simulink model "Vehicle_Model_999_Modular_roll_gradient"  (R2025b)
settings: Solver=ode23tb  StartTime=0.0  StopTime=30  MaxStep=0.001  RelTol=1e-3
values from neighbouring files (symbols this model uses):
  init_r = 0    [Run_this_first.m]
  init_vx = 0    [Run_this_first.m]
  init_vy = 0    [Run_this_first.m]
  Ki_array = zeros(size(Vx_array))    [Torque_vectoring_lookup_table_v3.m]    (also in Torque_vectoring_workspace_lookuptable_v2.m)
  Kp_array = zeros(size(Vx_array))    [Torque_vectoring_workspace_lookuptable_v2.m]
  ku = (lr*m/(cf*(lf+lr))) - (lf*m/(cr*(lf+lr)))    (= -0.000176093739153)    [Torque_vectoring_lookup_table_v3.m]    (also in Torque_vectoring_workspace_lookuptable_v2.m)
  m = Par.m    [LapSim_Endurance_final_ts_v2.m]    (also in Lap_Sim_Final_inverse.m = Par.Mass; Lapsim_Endurance_final_ts.m; New_LapSim_final_ts_v1.m = Par.Mass; Torque_vectoring_lookup_table_v3.m = 270)
  Par = struct()    [Load_vehicle_parameters.m]
  path_Theta = unwrap(atan2(dY, dX))    [New_LapSim_final_ts_v1.m]
  sus_par = struct()    [Load_sus_parameters.m]
  TireData = []    [Lapsim_final_for_app.m]
  V_ref = 45    [Run_this_first.m]
  Vx_array = 1:2:21    [Torque_vectoring_lookup_table_v3.m]    (also in Torque_vectoring_workspace_lookuptable_v2.m = 1:1:21)
undefined symbols (not defined in the file or in its folder): Battery, Brake_Val, ctrl_Brake, ctrl_s, ctrl_Steer, ctrl_Throttle, ctrl_Velocity, HP, Motor, path_X, path_Y, steer_input, Steer_Val, TC_target_slip, Throttle_Val
libraries: simulink x9, autolibshared x3, simulink_extras x2, BatteryEstimators x1
(part 2 of 4)

== system Vehicle_Model_999_Modular_roll_gradient/Vehicle dynamics/Rolling and Drag forces ==
  Aero Drag : MATLAB Function  TreatAsAtomicUnit=on
  Bus Creator : BusCreator  Inputs=3
  Bus Selector : BusSelector  OutputSignals=Fz
  Bus Selector1 : BusSelector  OutputSignals=Steer_FL,Steer_FR
  Bus Selector2 : BusSelector  OutputSignals=Longitudinal_vel,Lateral_vel
  MATLAB Function : MATLAB Function  TreatAsAtomicUnit=on
  Rolling Forces : MATLAB Function  TreatAsAtomicUnit=on
  Terminator : Terminator
  To Workspace : ToWorkspace  Commented=on  VariableName=Dragforce  SaveFormat=Timeseries  SampleTime=-1
  tag scope: Resistive_force_bus=global
  wires:
  Bus Selector1/1 -> Rolling Forces/2(Steer_FL)  "<Steer_FL>"
  Bus Selector2/1 -> Aero Drag/1(vx)  "<Longitudinal_vel>"
  Bus Selector/1 -> Rolling Forces/1(Fz)  "<Fz>"
  Aero Drag/1(B_F_aero) -> MATLAB Function/1(u), Bus Creator/3  "Aero_drag_force"
  Rolling Forces/1(Fx_rr_b) -> Bus Creator/1  "Longitudinal_rolling_resistance"
  Bus Selector1/2 -> Rolling Forces/3(Steer_FR)  "<Steer_FR>"
  Bus Selector2/2 -> Aero Drag/2(vy)  "<Lateral_vel>"
  Rolling Forces/2(Fy_rr_b) -> Bus Creator/2  "Lateral_rolling_resistance"
  Bus Creator/1 -> [Resistive_force_bus]
  MATLAB Function/1(y) -> To Workspace/1, Terminator/1  "Drag_force"
  [Wheel_bus] -> Bus Selector/1
  [Steer_bus] -> Bus Selector1/1
  [chassisbus] -> Bus Selector2/1

== system Vehicle_Model_999_Modular_roll_gradient/Vehicle dynamics/Steering ==
  Bus Selector12 : BusSelector  OutputSignals=Steer_input
  Constant1 : Constant  Value=sus_par.Acc_pct
  Steering Kinematics : Subsystem
  tag scope: Steer_bus=global
  wires:
  Bus Selector12/1 -> Steering Kinematics/1(Steer_Input)  "<Steer_input>"
  Constant1/1 -> Steering Kinematics/2(Ackermann_Pct)
  [Input_bus] -> Bus Selector12/1
  Steering Kinematics/1(Steering Angles) -> [Steer_bus]

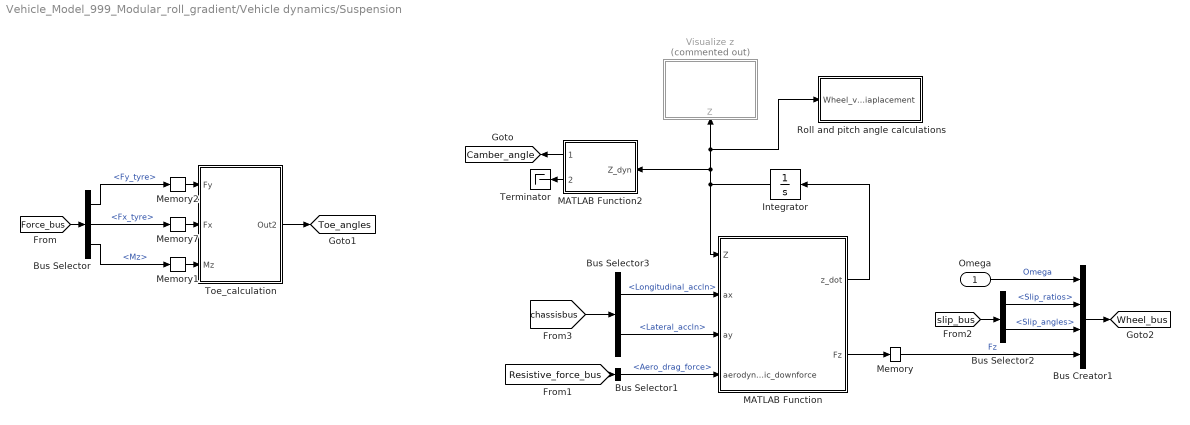
== system Vehicle_Model_999_Modular_roll_gradient/Vehicle dynamics/Suspension ==
  Omega : Inport
  Bus Creator1 : BusCreator  Inputs=4
  Bus Selector : BusSelector  OutputSignals=Fy_tyre,Fx_tyre,Mz
  Bus Selector1 : BusSelector  OutputSignals=Aero_drag_force
  Bus Selector2 : BusSelector  OutputSignals=Slip_ratios,Slip_angles
  Bus Selector3 : BusSelector  OutputSignals=Longitudinal_accln,Lateral_accln
  Integrator : Integrator
  MATLAB Function : MATLAB Function  TreatAsAtomicUnit=on
  MATLAB Function2 : MATLAB Function  TreatAsAtomicUnit=on
  Memory{,1..2,7} (4 alike) : Memory
  Roll and pitch angle calculations : Subsystem
  Terminator : Terminator
  Toe_calculation : Subsystem
  Visualize z : Subsystem  Commented=on
      settings: PortSchema="{\"entries\":[{\"content\":{\"sides\":[{\"content\":{},\"type\":\"ConnectorPlacement.EquallySpacedRectSide\",\"uuid\":\"aa7d9fe9-737c-43ef-afbb-9eca70b49cc7\"},{\"content\":{\"side\":\"RIGHT\"},\"type\":\"ConnectorPlacement.EquallySpacedRectSide\",\"uuid\":\"9d0ef4b4-3bdb-4078-8062-c9c6b9fc0eda\"},{\"content\":{\"side\":\"TOP\"},\"type\":\"ConnectorPlacement.EquallySpacedRectSide\",\"uuid\":\"423cb61c-0fc9-4741-ba0b-eea1eb6461c8\"},{\"content\":{\"connectorIds\":[\"In1\"],\"side\":\"BOTTOM\"},\"type\":\"ConnectorPlacement.EquallySpacedRectSide\",\"uuid\":\"d9a2c6e7-2104-49e5-8c96-ef23060413cc\"}]},\"type\":\"ConnectorPlacement.EquallySpacedConnector\",\"uuid\":\"46e784b7-ddd2-4d2c-b5cf-f45c70590aae\"}],\"packageUris\":[\"http://schema.mathworks.com/mf0/Connector/R2020b\"],\"version\":\"1.0\"}"
  tag scope: Camber_angle=global, Toe_angles=global, Wheel_bus=global
  wires:
  Toe_calculation/1(Out2) -> [Toe_angles]
  Memory7/1 -> Toe_calculation/2(Fx)
  Memory1/1 -> Toe_calculation/3(Mz)
  Memory2/1 -> Toe_calculation/1(Fy)
  Bus Selector/1 -> Memory2/1  "<Fy_tyre>"
  [Force_bus] -> Bus Selector/1
  Bus Selector/2 -> Memory7/1  "<Fx_tyre>"
  Bus Selector/3 -> Memory1/1  "<Mz>"
  Omega/1 -> Bus Creator1/1  "Omega"
  Bus Selector2/2 -> Bus Creator1/3  "<Slip_angles>"
  [chassisbus] -> Bus Selector3/1
  Bus Selector3/1 -> MATLAB Function/2(ax)  "<Longitudinal_accln>"
  Bus Selector2/1 -> Bus Creator1/2  "<Slip_ratios>"
  Bus Selector3/2 -> MATLAB Function/3(ay)  "<Lateral_accln>"
  MATLAB Function/1(z_dot) -> Integrator/1
  Bus Creator1/1 -> [Wheel_bus]
  [slip_bus] -> Bus Selector2/1
  Memory/1 -> Bus Creator1/4  "Fz"
  MATLAB Function/2(Fz) -> Memory/1
  Integrator/1 -> Roll and pitch angle calculations/1(Wheel_vertical_diaplacement), Visualize z/1(Z), MATLAB Function2/1(Z_dyn), MATLAB Function/1(Z)
  MATLAB Function2/1(Camber) -> [Camber_angle]
  MATLAB Function2/2(Camber_gain) -> Terminator/1
  [Resistive_force_bus] -> Bus Selector1/1
  Bus Selector1/1 -> MATLAB Function/4(aerodynamic_downforce)  "<Aero_drag_force>"

== system Vehicle_Model_999_Modular_roll_gradient/Vehicle dynamics/Wheel_dynamics ==
  Bus Selector13 : BusSelector  OutputSignals=Fz
  Bus Selector14 : BusSelector  OutputSignals=Slip_angles
  Bus Selector30 : BusSelector  OutputSignals=Omega
  Rolling Resistance : MATLAB Function  TreatAsAtomicUnit=on
  Wheel Dynamics : Subsystem
  Omega1 : Outport
  wires:
  [Wheel_bus] -> Bus Selector14/1, Bus Selector30/1, Bus Selector13/1
  Bus Selector30/1 -> Rolling Resistance/2(Omega)  "<Omega>"
  Rolling Resistance/1(wFx_rr) -> Wheel Dynamics/1(Fx_rr)
  Bus Selector13/1 -> Rolling Resistance/1(Fz)  "<Fz>"
  Bus Selector14/1 -> Rolling Resistance/3(slip_angles)  "<Slip_angles>"
  Wheel Dynamics/1(Omega) -> Omega1/1

== system Vehicle_Model_999_Modular_roll_gradient/Visualization/Visualize Fx ==
  Fx_tire : Inport
  Demux : Demux
  To Workspace : ToWorkspace  VariableName=Longitudinal_force_fl  SaveFormat=Timeseries  SampleTime=-1
  To Workspace1 : ToWorkspace  VariableName=Longitudinal_force_fr  SaveFormat=Timeseries  SampleTime=-1
  To Workspace2 : ToWorkspace  VariableName=Longitudinal_force_rl  SaveFormat=Timeseries  SampleTime=-1
  To Workspace3 : ToWorkspace  VariableName=Longitudinal_force_rr  SaveFormat=Timeseries  SampleTime=-1
  Visualize_longitudinal_force_tire : Scope  NumInputPorts=4
      settings: ActiveDisplayYMinimum=-1  ActiveDisplayYMaximum=1  DataLoggingVariableName=ScopeData2
  wires:
  Fx_tire/1 -> Demux/1
  Demux/1 -> To Workspace/1, Visualize_longitudinal_force_tire/1  "Longitudinal_force_fl"
  Demux/2 -> To Workspace1/1, Visualize_longitudinal_force_tire/2  "Longitudinal_force_fr"
  Demux/3 -> To Workspace2/1, Visualize_longitudinal_force_tire/3  "Longitudinal_force_rl"
  Demux/4 -> To Workspace3/1, Visualize_longitudinal_force_tire/4  "Longitudinal_force_rr"

== system Vehicle_Model_999_Modular_roll_gradient/Visualization/Visualize Fy ==
  Fy_tire : Inport
  Demux : Demux
  To Workspace1 : ToWorkspace  VariableName=Lateral_force_fl  SaveFormat=Timeseries  SampleTime=-1
  To Workspace2 : ToWorkspace  VariableName=Lateral_force_fr  SaveFormat=Timeseries  SampleTime=-1
  To Workspace3 : ToWorkspace  VariableName=Lateral_force_rl  SaveFormat=Timeseries  SampleTime=-1
  To Workspace4 : ToWorkspace  VariableName=Lateral_force_rr  SaveFormat=Timeseries  SampleTime=-1
  Visualize_lateral_force_tire : Scope  NumInputPorts=4
      settings: ActiveDisplayYMinimum=-1  ActiveDisplayYMaximum=1  DataLoggingVariableName=ScopeData2
  wires:
  Demux/4 -> To Workspace4/1, Visualize_lateral_force_tire/4  "Lateral_force_rr"
  Demux/3 -> To Workspace3/1, Visualize_lateral_force_tire/3  "Lateral_force_rl"
  Demux/2 -> To Workspace2/1, Visualize_lateral_force_tire/2  "Lateral_force_fr"
  Demux/1 -> To Workspace1/1, Visualize_lateral_force_tire/1  "Lateral_force_fl"
  Fy_tire/1 -> Demux/1

== system Vehicle_Model_999_Modular_roll_gradient/Visualization/Visualize Fz ==
  Fz : Inport
  Demux : Demux
  Visualize_Fz : Scope  NumInputPorts=4
      settings: ActiveDisplayYMinimum=-1  ActiveDisplayYMaximum=1  DataLoggingVariableName=ScopeData2
  wires:
  Fz/1 -> Demux/1
  Demux/1 -> Visualize_Fz/1  "Fz_fl"
  Demux/2 -> Visualize_Fz/2  "Fz_fr"
  Demux/3 -> Visualize_Fz/3  "Fz_rl"
  Demux/4 -> Visualize_Fz/4  "Fz_rr"

== system Vehicle_Model_999_Modular_roll_gradient/E-powertrain/Battery Pack/Subsystem ==
  In1 : Inport
  Constant : Constant  Value=0.001
  Switch : Switch  Criteria=u2 > Threshold  SaturateOnIntegerOverflow=off  InputSameDT=off
  Out1 : Outport
  wires:
  In1/1 -> Switch/1, Switch/2
  Constant/1 -> Switch/3
  Switch/1 -> Out1/1

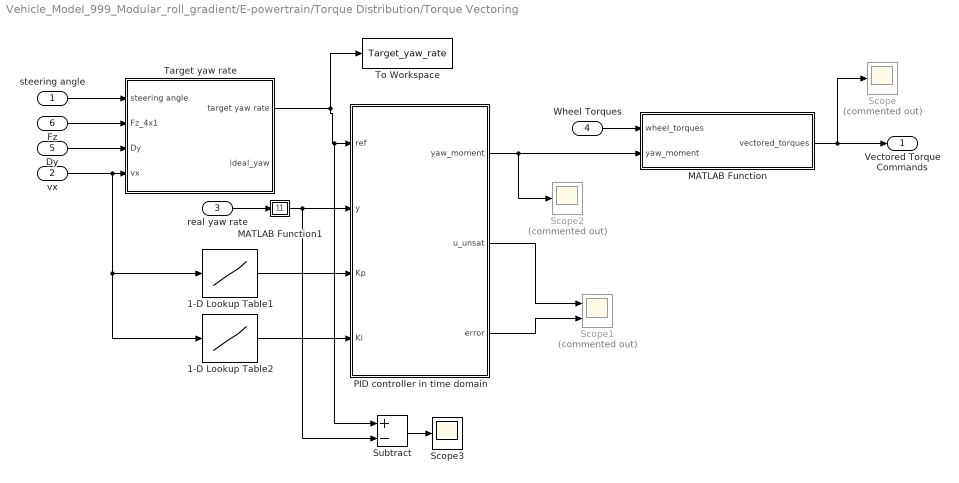
== system Vehicle_Model_999_Modular_roll_gradient/E-powertrain/Torque Distribution/Torque Vectoring ==
  steering angle : Inport
  vx : Inport  Port=2
  real yaw rate : Inport  Port=3
  Wheel Torques : Inport  Port=4
  Dy : Inport  Port=5
  Fz : Inport  Port=6
  1-D Lookup Table1 : Lookup_n-D  NumberOfTableDimensions=1  BreakpointsForDimension1=Vx_array  Table=Kp_array  InternalRulePriority=Speed  RndMeth=Simplest
  1-D Lookup Table2 : Lookup_n-D  NumberOfTableDimensions=1  BreakpointsForDimension1=Vx_array  Table=Ki_array  InternalRulePriority=Speed  RndMeth=Simplest
  MATLAB Function : MATLAB Function  TreatAsAtomicUnit=on
  MATLAB Function1 : MATLAB Function  TreatAsAtomicUnit=on
  PID controller in time domain : MATLAB Function  TreatAsAtomicUnit=on  SystemSampleTime=0.001
  Scope : Scope  Commented=on
      settings: ActiveDisplayYMinimum=-1  ActiveDisplayYMaximum=1  DataLoggingVariableName=ScopeData4
  Scope1 : Scope  Commented=on  NumInputPorts=2
      settings: ActiveDisplayYMinimum=-1  ActiveDisplayYMaximum=1  DataLoggingVariableName=ScopeData15
  Scope2 : Scope  Commented=on
      settings: ActiveDisplayYMinimum=-808.274340814801  ActiveDisplayYMaximum=139.13519650455567  DataLoggingVariableName=ScopeData17
  Scope3 : Scope
      settings: ActiveDisplayYMinimum=-0.85002897198767369  ActiveDisplayYMaximum=1.3983030281875917  DataLoggingVariableName=ScopeData18
  Subtract : Sum  Inputs=+-
  Target yaw rate : Subsystem
  To Workspace : ToWorkspace  VariableName=Target_yaw_rate  SaveFormat=Timeseries  SampleTime=-1
  Vectored Torque Commands : Outport
  wires:
  steering angle/1 -> Target yaw rate/1(steering angle)
  Wheel Torques/1 -> MATLAB Function/1(wheel_torques)
  MATLAB Function/1(vectored_torques) -> Scope/1, Vectored Torque Commands/1
  vx/1 -> 1-D Lookup Table2/1, 1-D Lookup Table1/1, Target yaw rate/4(vx)
  PID controller in time domain/1(yaw_moment) -> Scope2/1, MATLAB Function/2(yaw_moment)
  Fz/1 -> Target yaw rate/2(Fz_4x1)
  Dy/1 -> Target yaw rate/3(Dy)
  real yaw rate/1 -> MATLAB Function1/1(u)
  PID controller in time domain/2(u_unsat) -> Scope1/1
  PID controller in time domain/3(error) -> Scope1/2
  MATLAB Function1/1(y) -> Subtract/2, PID controller in time domain/2(y)
  1-D Lookup Table1/1 -> PID controller in time domain/3(Kp)
  1-D Lookup Table2/1 -> PID controller in time domain/4(Ki)
  Subtract/1 -> Scope3/1
  Target yaw rate/1(target yaw rate) -> Subtract/1, PID controller in time domain/1(ref), To Workspace/1

== system Vehicle_Model_999_Modular_roll_gradient/E-powertrain/Torque Distribution/Traction Control ==
  Wheel Torque : Inport
  Slip Ratios : Inport  Port=2
  vx : Inport  Port=3
  Constant3 : Constant  Value=TC_target_slip
  KD1 : Lookup_n-D  NumberOfTableDimensions=1  BreakpointsForDimension1=[0, 55e-10, 0.0045, 2, 8.5,9]  Table=[0, 0, 0.0014, 0.0109,0,0]  InternalRulePriority=Speed  RndMeth=Simplest
  KI1 : Lookup_n-D  NumberOfTableDimensions=1  BreakpointsForDimension1=[0; 55e-10;0.0045; 2; 8.5]  Table=[0.1; 0.1;700; 500; 450 ]  InternalRulePriority=Speed  RndMeth=Simplest
  KP1 : Lookup_n-D  NumberOfTableDimensions=1  BreakpointsForDimension1=[0; 55e-10; 0.0045; 2; 8.5]  Table=[ 0.5; 0.5; 2.5; 10; 10]  InternalRulePriority=Speed  RndMeth=Simplest
  MATLAB Function1 : MATLAB Function  TreatAsAtomicUnit=on  SystemSampleTime=0.001
  MATLAB Function2 : MATLAB Function  TreatAsAtomicUnit=on
  Traction Controlled Torque : Outport
  wires:
  KD1/1 -> MATLAB Function1/5(Kd)
  KI1/1 -> MATLAB Function1/4(Ki)
  KP1/1 -> MATLAB Function1/3(Kp)
  vx/1 -> KD1/1, KI1/1, KP1/1
  Slip Ratios/1 -> MATLAB Function1/2(lambda_actual)
  Constant3/1 -> MATLAB Function1/1(lambda_ref)
  Wheel Torque/1 -> MATLAB Function2/2(torque_wheel)
  MATLAB Function1/1(throttle_cmd) -> MATLAB Function2/1(torque_pid)
  MATLAB Function2/1(TC_output) -> Traction Controlled Torque/1

== system Vehicle_Model_999_Modular_roll_gradient/E-powertrain/Torque Distribution/is TCS on? ==
  traction_controlled_torque : Inport
  In1 : Inport  Port=2
  TV_T_wheel : Inport  Port=3
  AND : Logic  IconShape=distinctive  AllPortsSameDT=off  OutDataTypeStr=boolean
  NOT : Logic  Operator=NOT  IconShape=distinctive  AllPortsSameDT=off  OutDataTypeStr=boolean
  Switch : Switch  Criteria=u2 > Threshold  SaturateOnIntegerOverflow=off  InputSameDT=off
  torque_output : Outport
  wires:
  Switch/1 -> torque_output/1
  TV_T_wheel/1 -> Switch/3
  traction_controlled_torque/1 -> Switch/1
  In1/1 -> AND/2
  AND/1 -> Switch/2
  [Enable_TV] -> NOT/1
  NOT/1 -> AND/1

== system Vehicle_Model_999_Modular_roll_gradient/E-powertrain/Torque Distribution/is TV on? ==
  vectored_torque : Inport
  In1 : Inport  Port=2
  wheel_torque : Inport  Port=3
  AND : Logic  IconShape=distinctive  AllPortsSameDT=off  OutDataTypeStr=boolean
  Switch : Switch  Criteria=u2 > Threshold  SaturateOnIntegerOverflow=off  InputSameDT=off
  torque_output : Outport
  wires:
  wheel_torque/1 -> Switch/3
  vectored_torque/1 -> Switch/1
  Switch/1 -> torque_output/1
  AND/1 -> Switch/2
  In1/1 -> AND/2
  [Enable_TV] -> AND/1

== system Vehicle_Model_999_Modular_roll_gradient/Inputs/Brake_input_selector/Brake Variant Subsystem ==
  brake_sim : Inport
  vel : Inport  Port=2
  GGV : Subsystem  VariantControl=Mode_ggv
  Sideslip_vs_curvature_cst_accln : Subsystem  VariantControl=Mode_sideslip_vs_curvature_cst_accln
  Simulink : Subsystem  VariantControl=Mode_simulink
  curvature vs steer_angle : Subsystem  VariantControl=Mode_curvature_vs_steer
  sideslip_vs_curvature : Subsystem  VariantControl=Mode_sideslip_vs_curvature
  steerdiff_vs_ay : Subsystem  VariantControl=Mode_steerdiff_vs_ay
  timeseries : Subsystem  VariantControl=Mode_timeseries
  brake_input : Outport
  accln : Outport  Port=2

== system Vehicle_Model_999_Modular_roll_gradient/Inputs/Subsystem/Triggered Subsystem ==
  In1 : Inport
  Trigger : TriggerPort  VariantControl=(inherit)
  Out1 : Outport
  wires:
  In1/1 -> Out1/1

== system Vehicle_Model_999_Modular_roll_gradient/Inputs/Subsystem/Triggered Subsystem1 ==
  In1 : Inport
  Trigger : TriggerPort  VariantControl=(inherit)
  Out1 : Outport
  wires:
  In1/1 -> Out1/1

== system Vehicle_Model_999_Modular_roll_gradient/Inputs/Subsystem/Triggered Subsystem2 ==
  In1 : Inport
  Trigger : TriggerPort  VariantControl=(inherit)
  Out1 : Outport
  wires:
  In1/1 -> Out1/1

== system Vehicle_Model_999_Modular_roll_gradient/Inputs/Throttle_input_selector/Throttle Variant Subsystem ==
  accln : Inport
  accln_input_for_map1 : Inport  Port=2
  GGV : Subsystem  VariantControl=Mode_ggv
  Simulink : Subsystem  VariantControl=Mode_simulink
  Timeseries : Subsystem  VariantControl=Mode_timeseries
  curvature vs steer : Subsystem  VariantControl=Mode_curvature_vs_steer
  sideslip_vs_curvature : Subsystem  VariantControl=Mode_sideslip_vs_curvature
  sideslip_vs_curvature_cst_accln : Subsystem  VariantControl=Mode_sideslip_vs_curvature_cst_accln
  steerdiff_vs_ay : Subsystem  VariantControl=Mode_steerdiff_vs_ay
  throttle : Outport

== system Vehicle_Model_999_Modular_roll_gradient/Inputs/steer_input_selector/Steering Variant Subsystem ==
  In1 : Inport
  GGV : Subsystem  VariantControl=Mode_ggv
  Simulink : Subsystem  VariantControl=Mode_simulink
  Timeseries : Subsystem  VariantControl=Mode_timeseries
  curvature_vs_steering_angle : Subsystem  VariantControl=Mode_curvature_vs_steer
  sideslip_vs_curvature_1 : Subsystem  VariantControl=Mode_sideslip_vs_curvature
  sideslip_vs_curvature_constant_lat_accln : Subsystem  VariantControl=Mode_sideslip_vs_curvature_cst_accln
  steerdiff_vs_ay : Subsystem  VariantControl=Mode_steerdiff_vs_ay
  Steer Input : Outport

== system Vehicle_Model_999_Modular_roll_gradient/Vehicle dynamics/Force and Torque Equilibrium/Subsystem ==
  In1 : Inport
  Clock : Clock
  Compare To Constant : simulink/Logic and Bit Operations/Compare To Constant  relop=>=  const=75  OutDataTypeStr=boolean
  Detect Rise Positive : simulink/Logic and Bit Operations/Detect Rise Positive  vinit=0  OutDataTypeStr=boolean
  Triggered Subsystem : Subsystem  TreatAsAtomicUnit=on
  Out1 : Outport
  wires:
  In1/1 -> Compare To Constant/1
  Detect Rise Positive/1 -> Triggered Subsystem/Trigger
  Clock/1 -> Triggered Subsystem/1(In1)
  Triggered Subsystem/1(Out1) -> Out1/1
  Compare To Constant/1 -> Detect Rise Positive/1

== system Vehicle_Model_999_Modular_roll_gradient/Vehicle dynamics/Force and Torque Equilibrium/Subsystem1 ==
  In1 : Inport
  Constant : Constant  Value=0.001
  Switch : Switch  Criteria=u2 > Threshold  SaturateOnIntegerOverflow=off  InputSameDT=off
  Out1 : Outport
  wires:
  In1/1 -> Switch/1, Switch/2
  Constant/1 -> Switch/3
  Switch/1 -> Out1/1

== system Vehicle_Model_999_Modular_roll_gradient/Vehicle dynamics/Force and Torque Equilibrium/Visualize Fx ==
  Fx_body : Inport
  Demux : Demux
  To Workspace : ToWorkspace  VariableName=Longitudinal_force_body_fl  SaveFormat=Timeseries  SampleTime=-1
  To Workspace1 : ToWorkspace  VariableName=Longitudinal_force_body_fr  SaveFormat=Timeseries  SampleTime=-1
  To Workspace2 : ToWorkspace  VariableName=Longitudinal_force_body_rl  SaveFormat=Timeseries  SampleTime=-1
  To Workspace3 : ToWorkspace  VariableName=Longitudinal_force_body_rr  SaveFormat=Timeseries  SampleTime=-1
  Visualize_longitudinal_force_body : Scope  NumInputPorts=4
      settings: ActiveDisplayYMinimum=-1  ActiveDisplayYMaximum=1  DataLoggingVariableName=ScopeData2
  wires:
  Fx_body/1 -> Demux/1
  Demux/1 -> To Workspace/1, Visualize_longitudinal_force_body/1  "Longitudinal_force_fl"
  Demux/2 -> To Workspace1/1, Visualize_longitudinal_force_body/2  "Longitudinal_force_fr"
  Demux/3 -> To Workspace2/1, Visualize_longitudinal_force_body/3  "Longitudinal_force_rl"
  Demux/4 -> To Workspace3/1, Visualize_longitudinal_force_body/4  "Longitudinal_force_rr"

== system Vehicle_Model_999_Modular_roll_gradient/Vehicle dynamics/Force and Torque Equilibrium/Visualize Fy ==
  Fy_tire : Inport
  Demux : Demux
  To Workspace1 : ToWorkspace  VariableName=Lateral_force_body_fl  SaveFormat=Timeseries  SampleTime=-1
  To Workspace2 : ToWorkspace  VariableName=Lateral_force_body_fr  SaveFormat=Timeseries  SampleTime=-1
  To Workspace3 : ToWorkspace  VariableName=Lateral_force_body_rl  SaveFormat=Timeseries  SampleTime=-1
  To Workspace4 : ToWorkspace  VariableName=Lateral_force_body_rr  SaveFormat=Timeseries  SampleTime=-1
  Visualize_lateral_force_body : Scope  NumInputPorts=4
      settings: ActiveDisplayYMinimum=-1  ActiveDisplayYMaximum=1  DataLoggingVariableName=ScopeData2
  wires:
  Demux/4 -> To Workspace4/1, Visualize_lateral_force_body/4  "Lateral_force_rr"
  Demux/3 -> To Workspace3/1, Visualize_lateral_force_body/3  "Lateral_force_rl"
  Demux/2 -> To Workspace2/1, Visualize_lateral_force_body/2  "Lateral_force_fr"
  Demux/1 -> To Workspace1/1, Visualize_lateral_force_body/1  "Lateral_force_fl"
  Fy_tire/1 -> Demux/1

== system Vehicle_Model_999_Modular_roll_gradient/Vehicle dynamics/Fx, Fy calculations/Slip_angle_calculation ==
  Bus Selector25 : BusSelector  OutputSignals=Longitudinal_vel
  Bus Selector26 : BusSelector  OutputSignals=Lateral_vel
  Bus Selector27 : BusSelector  OutputSignals=Yaw_rate
  Bus Selector28 : BusSelector  OutputSignals=Steer_FL
  Bus Selector29 : BusSelector  OutputSignals=Steer_FR
  Slip Angles : MATLAB Function  TreatAsAtomicUnit=on
  Subsystem : Subsystem
  Visualize Slip_angle : Subsystem  Commented=on
  effective_slip_angle : Outport
  wires:
  Bus Selector26/1 -> Slip Angles/2(Lateral_vel)  "<Lateral_vel>"
  Bus Selector27/1 -> Slip Angles/3(yawrate)  "<Yaw_rate>"
  [Steer_bus] -> Bus Selector29/1, Bus Selector28/1
  [chassisbus] -> Bus Selector27/1, Bus Selector26/1, Bus Selector25/1
  Bus Selector25/1 -> Slip Angles/1(Longitudinal_vel)  "<Longitudinal_vel>"
  Slip Angles/1(slip_angles) -> Subsystem/2(slip_angles)
  Bus Selector28/1 -> Slip Angles/4(Steer_FL)  "<Steer_FL>"
  Bus Selector29/1 -> Slip Angles/5(Steer_FR)  "<Steer_FR>"
  Subsystem/1(slip_ratio) -> Visualize Slip_angle/1(slip_angle), effective_slip_angle/1  "effective_slip_angle"
  [Toe_angles] -> Subsystem/1(toe)

== system Vehicle_Model_999_Modular_roll_gradient/Vehicle dynamics/Fx, Fy calculations/Slip_ratio_calculation ==
  Bus Selector21 : BusSelector  OutputSignals=Longitudinal_vel
  Bus Selector22 : BusSelector  OutputSignals=Yaw_rate
  Bus Selector23 : BusSelector  OutputSignals=Omega
  Bus Selector24 : BusSelector  OutputSignals=Lateral_vel
  Bus Selector32 : BusSelector  OutputSignals=Steer_FL
  Bus Selector33 : BusSelector  OutputSignals=Steer_FR
  Visualize Slip_ratios : Subsystem  Commented=on
  slip ratios : MATLAB Function  TreatAsAtomicUnit=on
  slip_ratios : Outport
  wires:
  [Steer_bus] -> Bus Selector32/1, Bus Selector33/1
  Bus Selector21/1 -> slip ratios/1(Vx)  "<Longitudinal_vel>"
  Bus Selector23/1 -> slip ratios/4(Omega)  "<Omega>"
  Bus Selector32/1 -> slip ratios/5(Steer_FL)  "<Steer_FL>"
  [chassisbus] -> Bus Selector22/1, Bus Selector24/1, Bus Selector21/1
  Bus Selector22/1 -> slip ratios/3(yawrate)  "<Yaw_rate>"
  Bus Selector33/1 -> slip ratios/6(Steer_FR)  "<Steer_FR>"
  Bus Selector24/1 -> slip ratios/2(Vy)  "<Lateral_vel>"
  [Wheel_bus] -> Bus Selector23/1
  slip ratios/1(slip_ratios) -> Visualize Slip_ratios/1(slip_ratio), slip_ratios/1  "slip_ratios"

== system Vehicle_Model_999_Modular_roll_gradient/Vehicle dynamics/Fx, Fy calculations/Tyre_relaxation ==
  Fx_ss : Inport
  Bus Selector : BusSelector  OutputSignals=Longitudinal_vel
  Integrator : Integrator
  MATLAB Function : MATLAB Function  TreatAsAtomicUnit=on
  Fx_w : Outport
  wires:
  Fx_ss/1 -> MATLAB Function/1(Fx_ss)
  MATLAB Function/1(Fx_dot) -> Integrator/1
  Integrator/1 -> Fx_w/1, MATLAB Function/2(Fx_act)
  Bus Selector/1 -> MATLAB Function/3(Vx)  "<Longitudinal_vel>"
  [chassisbus] -> Bus Selector/1

== system Vehicle_Model_999_Modular_roll_gradient/Vehicle dynamics/Fx, Fy calculations/Visualise_Fy_B ==
  Fy_B : Inport
  MATLAB Function : MATLAB Function  TreatAsAtomicUnit=on
  Visualise Fy_B : Scope  Commented=on  NumInputPorts=4
  wires:
  Fy_B/1 -> MATLAB Function/1(Fy_tire)
  MATLAB Function/2(Fy_B_fr) -> Visualise Fy_B/2  "Fy_B_fr"
  MATLAB Function/4(Fy_B_rr) -> Visualise Fy_B/4  "Fy_B_rr"
  MATLAB Function/1(Fy_B_fl) -> Visualise Fy_B/1  "Fy_B_fl"
  MATLAB Function/3(Fy_B_rl) -> Visualise Fy_B/3  "Fy_B_rl"

== system Vehicle_Model_999_Modular_roll_gradient/Vehicle dynamics/Fx, Fy calculations/Visualiser ==
  mz : Inport
  mu_x : Inport  Port=2
  mu_y : Inport  Port=3
  Demux : Demux
  Demux1 : Demux
  Demux2 : Demux
  Scope : Scope  NumInputPorts=4
  Scope1 : Scope  NumInputPorts=4
  Scope2 : Scope  NumInputPorts=4
  wires:
  mz/1 -> Demux/1
  Demux/1 -> Scope/1
  Demux/2 -> Scope/2
  Demux/3 -> Scope/3
  Demux/4 -> Scope/4
  Demux1/3 -> Scope1/3
  Demux1/2 -> Scope1/2
  mu_x/1 -> Demux1/1
  Demux1/1 -> Scope1/1
  Demux1/4 -> Scope1/4
  Demux2/3 -> Scope2/3
  Demux2/2 -> Scope2/2
  mu_y/1 -> Demux2/1
  Demux2/1 -> Scope2/1
  Demux2/4 -> Scope2/4

== system Vehicle_Model_999_Modular_roll_gradient/Vehicle dynamics/Fx, Fy calculations with grip limit/Grip_limit ==
  Fx : Inport
  Fy_tyre : Inport  Port=2
  Bus Selector2 : BusSelector  OutputSignals=Dx,Dy
  Bus Selector3 : BusSelector  OutputSignals=Longitudinal_disp
  MATLAB Function1 : MATLAB Function  TreatAsAtomicUnit=on
  Fx_new : Outport
  Fy_new : Outport  Port=2
  wires:
  Bus Selector2/2 -> MATLAB Function1/4(Dy)  "<Dy>"
  Bus Selector3/1 -> MATLAB Function1/5(s)  "<Longitudinal_disp>"
  Bus Selector2/1 -> MATLAB Function1/3(Dx)  "<Dx>"
  [chassisbus] -> Bus Selector3/1
  [Force_bus] -> Bus Selector2/1
  MATLAB Function1/1(Fx_new) -> Fx_new/1
  Fy_tyre/1 -> MATLAB Function1/2(Fy)
  Fx/1 -> MATLAB Function1/1(Fx)
  MATLAB Function1/2(Fy_new) -> Fy_new/1

== system Vehicle_Model_999_Modular_roll_gradient/Vehicle dynamics/Fx, Fy calculations with grip limit/Slip_angle_calculation ==
  Bus Selector25 : BusSelector  OutputSignals=Longitudinal_vel
  Bus Selector26 : BusSelector  OutputSignals=Lateral_vel
  Bus Selector27 : BusSelector  OutputSignals=Yaw_rate
  Bus Selector28 : BusSelector  OutputSignals=Steer_FL
  Bus Selector29 : BusSelector  OutputSignals=Steer_FR
  Slip Angles : MATLAB Function  TreatAsAtomicUnit=on
  Subsystem : Subsystem
  Visualize Slip_angle : Subsystem  Commented=on
  effective_slip_angle : Outport
  wires:
  [Toe_angles] -> Subsystem/1(toe)
  Subsystem/1(slip_ratio) -> effective_slip_angle/1, Visualize Slip_angle/1(slip_angle)  "effective_slip_angle"
  Bus Selector29/1 -> Slip Angles/5(Steer_FR)  "<Steer_FR>"
  Bus Selector28/1 -> Slip Angles/4(Steer_FL)  "<Steer_FL>"
  Slip Angles/1(slip_angles) -> Subsystem/2(slip_angles)
  Bus Selector25/1 -> Slip Angles/1(Longitudinal_vel)  "<Longitudinal_vel>"
  [chassisbus] -> Bus Selector25/1, Bus Selector26/1, Bus Selector27/1
  [Steer_bus] -> Bus Selector28/1, Bus Selector29/1
  Bus Selector27/1 -> Slip Angles/3(yawrate)  "<Yaw_rate>"
  Bus Selector26/1 -> Slip Angles/2(Lateral_vel)  "<Lateral_vel>"

== system Vehicle_Model_999_Modular_roll_gradient/Vehicle dynamics/Fx, Fy calculations with grip limit/Slip_ratio_calculation ==
  Bus Selector21 : BusSelector  OutputSignals=Longitudinal_vel
  Bus Selector22 : BusSelector  OutputSignals=Yaw_rate
  Bus Selector23 : BusSelector  OutputSignals=Omega
  Bus Selector24 : BusSelector  OutputSignals=Lateral_vel
  Bus Selector32 : BusSelector  OutputSignals=Steer_FL
  Bus Selector33 : BusSelector  OutputSignals=Steer_FR
  Visualize Slip_ratios : Subsystem  Commented=on
  slip ratios : MATLAB Function  TreatAsAtomicUnit=on
  slip_ratios : Outport
  wires:
  slip ratios/1(slip_ratios) -> slip_ratios/1, Visualize Slip_ratios/1(slip_ratio)  "slip_ratios"
  [Wheel_bus] -> Bus Selector23/1
  Bus Selector24/1 -> slip ratios/2(Vy)  "<Lateral_vel>"
  Bus Selector33/1 -> slip ratios/6(Steer_FR)  "<Steer_FR>"
  Bus Selector22/1 -> slip ratios/3(yawrate)  "<Yaw_rate>"
  [chassisbus] -> Bus Selector21/1, Bus Selector24/1, Bus Selector22/1
  Bus Selector32/1 -> slip ratios/5(Steer_FL)  "<Steer_FL>"
  Bus Selector23/1 -> slip ratios/4(Omega)  "<Omega>"
  Bus Selector21/1 -> slip ratios/1(Vx)  "<Longitudinal_vel>"
  [Steer_bus] -> Bus Selector33/1, Bus Selector32/1

== system Vehicle_Model_999_Modular_roll_gradient/Vehicle dynamics/Fx, Fy calculations with grip limit/Tyre_relaxation ==
  Fx_ss : Inport
  Bus Selector : BusSelector  OutputSignals=Longitudinal_vel
  Integrator : Integrator
  MATLAB Function : MATLAB Function  TreatAsAtomicUnit=on
  Fx_w : Outport
  wires:
  [chassisbus] -> Bus Selector/1
  Bus Selector/1 -> MATLAB Function/3(Vx)  "<Longitudinal_vel>"
  Integrator/1 -> MATLAB Function/2(Fx_act), Fx_w/1
  MATLAB Function/1(Fx_dot) -> Integrator/1
  Fx_ss/1 -> MATLAB Function/1(Fx_ss)

== system Vehicle_Model_999_Modular_roll_gradient/Vehicle dynamics/Fx, Fy calculations with grip limit/Visualise_Fy_B ==
  Fy_B : Inport
  MATLAB Function : MATLAB Function  TreatAsAtomicUnit=on
  Visualise Fy_B : Scope  Commented=on  NumInputPorts=4
  wires:
  MATLAB Function/3(Fy_B_rl) -> Visualise Fy_B/3  "Fy_B_rl"
  MATLAB Function/1(Fy_B_fl) -> Visualise Fy_B/1  "Fy_B_fl"
  MATLAB Function/4(Fy_B_rr) -> Visualise Fy_B/4  "Fy_B_rr"
  MATLAB Function/2(Fy_B_fr) -> Visualise Fy_B/2  "Fy_B_fr"
  Fy_B/1 -> MATLAB Function/1(Fy_tire)

== system Vehicle_Model_999_Modular_roll_gradient/Vehicle dynamics/Fx, Fy calculations with grip limit/Visualiser ==
  mz : Inport
  mu_x : Inport  Port=2
  mu_y : Inport  Port=3
  Demux : Demux
  Demux1 : Demux
  Demux2 : Demux
  Scope : Scope  NumInputPorts=4
  Scope1 : Scope  NumInputPorts=4
  Scope2 : Scope  NumInputPorts=4
  wires:
  Demux2/4 -> Scope2/4
  Demux2/1 -> Scope2/1
  mu_y/1 -> Demux2/1
  Demux2/2 -> Scope2/2
  Demux2/3 -> Scope2/3
  Demux1/4 -> Scope1/4
  Demux1/1 -> Scope1/1
  mu_x/1 -> Demux1/1
  Demux1/2 -> Scope1/2
  Demux1/3 -> Scope1/3
  Demux/4 -> Scope/4
  Demux/3 -> Scope/3
  Demux/2 -> Scope/2
  Demux/1 -> Scope/1
  mz/1 -> Demux/1

== system Vehicle_Model_999_Modular_roll_gradient/Vehicle dynamics/Steering/Steering Kinematics ==
  Steer_Input : Inport
  Ackermann_Pct : Inport  Port=2
  Bus Creator1 : BusCreator  Inputs=2
  Steering Kinematics : MATLAB Function  TreatAsAtomicUnit=on
  To Workspace : ToWorkspace  VariableName=steer_L  SaveFormat=Timeseries  SampleTime=-1
  To Workspace1 : ToWorkspace  VariableName=steer_R  SaveFormat=Timeseries  SampleTime=-1
  Steering Angles : Outport
  wires:
  Steering Kinematics/1(Steer_FL) -> To Workspace/1, Bus Creator1/1  "Steer_FL"
  Steer_Input/1 -> Steering Kinematics/1(Steer_Input)
  Steering Kinematics/2(Steer_FR) -> To Workspace1/1, Bus Creator1/2  "Steer_FR"
  Ackermann_Pct/1 -> Steering Kinematics/2(Ackermann_Pct)
  Bus Creator1/1 -> Steering Angles/1

== system Vehicle_Model_999_Modular_roll_gradient/Vehicle dynamics/Suspension/Roll and pitch angle calculations ==
  Wheel_vertical_diaplacement : Inport
  Gain : Gain  Gain=180/pi
  Gain1 : Gain  Gain=180/pi
  Pitch_angle_calcualtions : MATLAB Function  TreatAsAtomicUnit=on
  Roll_angle_calulations : MATLAB Function  TreatAsAtomicUnit=on
  To Workspace : ToWorkspace  VariableName=roll_angle  SaveFormat=Timeseries  SampleTime=-1
  Visualize pitch angle : Scope
      settings: ActiveDisplayYMinimum=-0.081148408984306142  ActiveDisplayYMaximum=0.65312774588570066  DataLoggingVariableName=ScopeData5
  Visualize roll angle : Scope
      settings: ActiveDisplayYMinimum=-1  ActiveDisplayYMaximum=1  DataLoggingVariableName=ScopeData6
  wires:
  Wheel_vertical_diaplacement/1 -> Pitch_angle_calcualtions/1(z_wheel), Roll_angle_calulations/1(z_wheel)
  Pitch_angle_calcualtions/1(Pitch_angle) -> Gain/1
  Roll_angle_calulations/1(Roll_angle) -> Gain1/1
  Gain/1 -> Visualize pitch angle/1
  Gain1/1 -> To Workspace/1, Visualize roll angle/1

== system Vehicle_Model_999_Modular_roll_gradient/Vehicle dynamics/Suspension/Toe_calculation ==
  Fy : Inport
  Fx : Inport  Port=2
  Mz : Inport  Port=3
  Mux1 : Mux
  toe_fl1 : MATLAB Function  TreatAsAtomicUnit=on
  Out2 : Outport
  wires:
  Mux1/1 -> Out2/1
  Mz/1 -> toe_fl1/3(Mz)
  Fx/1 -> toe_fl1/2(Fx_tire)
  Fy/1 -> toe_fl1/1(Fy_tire)
  toe_fl1/1(Toe_fl) -> Mux1/1
  toe_fl1/2(Toe_fr) -> Mux1/2
  toe_fl1/3(Toe_rl) -> Mux1/3
  toe_fl1/4(Toe_rr) -> Mux1/4

== system Vehicle_Model_999_Modular_roll_gradient/Vehicle dynamics/Suspension/Visualize z ==
  Z : Inport
  Demux : Demux
  Visualize_wheel_vertical_displacement : Scope  NumInputPorts=4
      settings: ActiveDisplayYMinimum=-0.0083526738061748679  ActiveDisplayYMaximum=0.0034975178963681597  DataLoggingVariableName=ScopeData2
  wires:
  Z/1 -> Demux/1
  Demux/1 -> Visualize_wheel_vertical_displacement/1  "z_fl"
  Demux/2 -> Visualize_wheel_vertical_displacement/2  "z_fr"
  Demux/3 -> Visualize_wheel_vertical_displacement/3  "z_rl"
  Demux/4 -> Visualize_wheel_vertical_displacement/4  "z_rr"

== system Vehicle_Model_999_Modular_roll_gradient/Vehicle dynamics/Wheel_dynamics/Wheel Dynamics ==
  Fx_rr : Inport
  Bus Selector8 : BusSelector  OutputSignals=Fx_tyre
  Integrator : Integrator  InitialCondition=init_vx/Par.R0  LimitOutput=on  UpperSaturationLimit=1e6
  MATLAB Function : MATLAB Function  TreatAsAtomicUnit=on
  Saturation : Saturate  UpperLimit=Motor.n_max*2*pi/(60*10.05)  LowerLimit=0
  Omega : Outport
  wires:
  [Torque_inputs] -> MATLAB Function/1(T_in)
  Fx_rr/1 -> MATLAB Function/2(Fx_rr)
  Integrator/1 -> Saturation/1
  MATLAB Function/1(Omega_dot) -> Integrator/1
  [Force_bus] -> Bus Selector8/1
  Bus Selector8/1 -> MATLAB Function/3(Fx_tire)  "<Fx_tyre>"
  Saturation/1 -> Omega/1, MATLAB Function/4(Omega)

== system Vehicle_Model_999_Modular_roll_gradient/E-powertrain/Torque Distribution/Torque Vectoring/Target yaw rate ==
  steering angle : Inport
  Fz_4x1 : Inport  Port=2
  Dy : Inport  Port=3
  vx : Inport  Port=4
  MATLAB Function : MATLAB Function  TreatAsAtomicUnit=on
  target yaw rate : Outport
  ideal_yaw : Outport  Port=2
  tag scope: Enable_TV=global
  wires:
  vx/1 -> MATLAB Function/1(vx)
  Fz_4x1/1 -> MATLAB Function/4(Fz)
  Dy/1 -> MATLAB Function/3(Dy)
  steering angle/1 -> MATLAB Function/2(delta)
  MATLAB Function/1(target_yaw) -> target yaw rate/1
  MATLAB Function/2(ideal_yaw) -> ideal_yaw/1
  MATLAB Function/3(tv_enable) -> [Enable_TV]

== system Vehicle_Model_999_Modular_roll_gradient/Inputs/Brake_input_selector/Brake Variant Subsystem/GGV ==
  Constant : Constant  Value=Brake_Val
  brake_input : Outport
  wires:
  Constant/1 -> brake_input/1

== system Vehicle_Model_999_Modular_roll_gradient/Inputs/Brake_input_selector/Brake Variant Subsystem/Sideslip_vs_curvature_cst_accln ==
  vel : Inport
  Constant : Constant  Value=10
  Constant3 : Constant  Value=0
  Longitudinal Driver : autolibshared/Longitudinal Driver  extAccelOvr=off  extDecelOvr=off  extAccelHld=off  extDecelHld=off  extAccelZero=off  extDecelZero=off  cntrlType=PI  shftType=None  velUnits=m/s  gearOut=off  Kp=10  Ki=5  Kff=.1  Kg=0  VehVelVec=[0 100]  KffVec=[.1 .1]  KpVec=[10 10]  KiVec=[5 5]  KgVec=[0 0]  m=1500  Kpt=3000  tau=.1  L=2  aR=200  bR=2.5  cR=.5  g=9.81  vnom=5  Kaw=1  tauerr=.01  tauPt=2  GearInit=0  tShift=.1  pdlVec=[0.1 0.4 0.5 0.9]  upShftTbl=[-1 12.9375 26.4375 39.9375 51.18749999999999 62.4375 72.84375 83.25;-1 16.3125 29.8125 43.3125 54.5624 65.8125 76.78125 87.75;-1 19.6875 33.1875 46.68749999999999 57.9375 69.1875 80.71875 92.25;-1 33 52.5 77.25 100.5 138.75 161.875 185]  dwnShftTbl=[1 9.5625 23.0625 36.5625 47.8125 59.0625 68.90625 78.75;1 12.9375 26.4375 39.9375 51.18749999999999 62.4375 72.84375 83.25;1 16.3125 29.8125 43.3125 54.562499 65.8125 76.78125 87.75;1 19.6875 33.1875 46.68749999999999 57.9375 69.1875 80.71875 92.25]  tClutch=.5  tRev=.5  tPark=120  aMode=2  UpGearVec="[0  1  2  3  4  5  6  7]"  DownGearVec="[1  2  3  4  5  6  7  8]"
      settings: LibrarySourceBlock=vehdynlibdriver/Longitudinal Driver
  Terminator1 : Terminator
  brake_input : Outport
  accln : Outport  Port=2
  wires:
  Constant3/1 -> Longitudinal Driver/3
  Constant/1 -> Longitudinal Driver/1
  Longitudinal Driver/1 -> Terminator1/1
  Longitudinal Driver/2 -> accln/1
  Longitudinal Driver/3 -> brake_input/1
  vel/1 -> Longitudinal Driver/2

== system Vehicle_Model_999_Modular_roll_gradient/Inputs/Brake_input_selector/Brake Variant Subsystem/Simulink ==
  brake_sim : Inport
  brake_input : Outport
  wires:
  brake_sim/1 -> brake_input/1

== system Vehicle_Model_999_Modular_roll_gradient/Inputs/Brake_input_selector/Brake Variant Subsystem/curvature vs steer_angle ==
  vel : Inport
  Constant : Constant  Value=V_ref
  Constant3 : Constant  Value=0
  Longitudinal Driver : autolibshared/Longitudinal Driver  extAccelOvr=off  extDecelOvr=off  extAccelHld=off  extDecelHld=off  extAccelZero=off  extDecelZero=off  cntrlType=PI  shftType=None  velUnits=m/s  gearOut=off  Kp=10  Ki=5  Kff=.1  Kg=0  VehVelVec=[0 100]  KffVec=[.1 .1]  KpVec=[10 10]  KiVec=[5 5]  KgVec=[0 0]  m=1500  Kpt=3000  tau=.1  L=2  aR=200  bR=2.5  cR=.5  g=9.81  vnom=5  Kaw=1  tauerr=.01  tauPt=2  GearInit=0  tShift=.1  pdlVec=[0.1 0.4 0.5 0.9]  upShftTbl=[-1 12.9375 26.4375 39.9375 51.18749999999999 62.4375 72.84375 83.25;-1 16.3125 29.8125 43.3125 54.5624 65.8125 76.78125 87.75;-1 19.6875 33.1875 46.68749999999999 57.9375 69.1875 80.71875 92.25;-1 33 52.5 77.25 100.5 138.75 161.875 185]  dwnShftTbl=[1 9.5625 23.0625 36.5625 47.8125 59.0625 68.90625 78.75;1 12.9375 26.4375 39.9375 51.18749999999999 62.4375 72.84375 83.25;1 16.3125 29.8125 43.3125 54.562499 65.8125 76.78125 87.75;1 19.6875 33.1875 46.68749999999999 57.9375 69.1875 80.71875 92.25]  tClutch=.5  tRev=.5  tPark=120  aMode=2  UpGearVec="[0  1  2  3  4  5  6  7]"  DownGearVec="[1  2  3  4  5  6  7  8]"
      settings: LibrarySourceBlock=vehdynlibdriver/Longitudinal Driver
  Terminator : Terminator
  brake_input : Outport
  accln : Outport  Port=2
  wires:
  Longitudinal Driver/3 -> brake_input/1
  Constant3/1 -> Longitudinal Driver/3
  Longitudinal Driver/1 -> Terminator/1
  Constant/1 -> Longitudinal Driver/1
  Longitudinal Driver/2 -> accln/1
  vel/1 -> Longitudinal Driver/2

== system Vehicle_Model_999_Modular_roll_gradient/Inputs/Brake_input_selector/Brake Variant Subsystem/sideslip_vs_curvature ==
  brake_sim : Inport
  brake_input : Outport
  wires:
  brake_sim/1 -> brake_input/1

== system Vehicle_Model_999_Modular_roll_gradient/Inputs/Brake_input_selector/Brake Variant Subsystem/steerdiff_vs_ay ==
  Constant : Constant  Value=0
  brake_input : Outport
  wires:
  Constant/1 -> brake_input/1

== system Vehicle_Model_999_Modular_roll_gradient/Inputs/Brake_input_selector/Brake Variant Subsystem/timeseries ==
  From Workspace : FromWorkspace  VariableName=brake_ts
  brake_input : Outport
  wires:
  From Workspace/1 -> brake_input/1

== system Vehicle_Model_999_Modular_roll_gradient/Inputs/Throttle_input_selector/Throttle Variant Subsystem/GGV ==
  SimInput_Throttle : Constant  Value=Throttle_Val
  throttle : Outport
  wires:
  SimInput_Throttle/1 -> throttle/1

== system Vehicle_Model_999_Modular_roll_gradient/Inputs/Throttle_input_selector/Throttle Variant Subsystem/Simulink ==
  accln : Inport
  throttle : Outport
  wires:
  accln/1 -> throttle/1

== system Vehicle_Model_999_Modular_roll_gradient/Inputs/Throttle_input_selector/Throttle Variant Subsystem/Timeseries ==
  From Workspace : FromWorkspace  VariableName=throttle_ts
  throttle : Outport
  wires:
  From Workspace/1 -> throttle/1

== system Vehicle_Model_999_Modular_roll_gradient/Inputs/Throttle_input_selector/Throttle Variant Subsystem/curvature vs steer ==
  accln_input_for_map1 : Inport
  throttle : Outport
  wires:
  accln_input_for_map1/1 -> throttle/1

== system Vehicle_Model_999_Modular_roll_gradient/Inputs/Throttle_input_selector/Throttle Variant Subsystem/sideslip_vs_curvature ==
  Constant : Constant
  throttle : Outport
  wires:
  Constant/1 -> throttle/1

== system Vehicle_Model_999_Modular_roll_gradient/Inputs/Throttle_input_selector/Throttle Variant Subsystem/sideslip_vs_curvature_cst_accln ==
  accln_input_for_map1 : Inport
  throttle : Outport
  wires:
  accln_input_for_map1/1 -> throttle/1

== system Vehicle_Model_999_Modular_roll_gradient/Inputs/Throttle_input_selector/Throttle Variant Subsystem/steerdiff_vs_ay ==
  Clock : Clock
  Constant1 : Constant  Value=0.25
  Ramp : simulink/Sources/Ramp  slope=2  start=0  InitialOutput=0
  Saturation : Saturate  UpperLimit=1  LowerLimit=0
  Switch : Switch  Criteria=u2 > Threshold  Threshold=4  SaturateOnIntegerOverflow=off  InputSameDT=off
  throttle : Outport
  wires:
  Clock/1 -> Switch/2
  Ramp/1 -> Switch/3
  Switch/1 -> Saturation/1
  Constant1/1 -> Switch/1
  Saturation/1 -> throttle/1

== system Vehicle_Model_999_Modular_roll_gradient/Inputs/steer_input_selector/Steering Variant Subsystem/GGV ==
  SimInput_Steer : Constant  Value=Steer_Val
  Steer Input : Outport
  wires:
  SimInput_Steer/1 -> Steer Input/1

== system Vehicle_Model_999_Modular_roll_gradient/Inputs/steer_input_selector/Steering Variant Subsystem/Simulink ==
  In1 : Inport
  Steer Input : Outport
  wires:
  In1/1 -> Steer Input/1

== system Vehicle_Model_999_Modular_roll_gradient/Inputs/steer_input_selector/Steering Variant Subsystem/Timeseries ==
  From Workspace : FromWorkspace  VariableName=steer_ts
  Steer Input : Outport
  wires:
  From Workspace/1 -> Steer Input/1

== system Vehicle_Model_999_Modular_roll_gradient/Inputs/steer_input_selector/Steering Variant Subsystem/curvature_vs_steering_angle ==
  Clock1 : Clock
  Constant1 : Constant  Value=0
  Ramp2 : simulink/Sources/Ramp  slope=pi/60  start=10  InitialOutput=0
  Saturation1 : Saturate  UpperLimit=pi/6
  Switch1 : Switch  Criteria=u2 > Threshold  Threshold=10  SaturateOnIntegerOverflow=off  InputSameDT=off
  Steer Input : Outport
  wires:
  Switch1/1 -> Saturation1/1
  Ramp2/1 -> Switch1/1
  Clock1/1 -> Switch1/2
  Constant1/1 -> Switch1/3
  Saturation1/1 -> Steer Input/1

== system Vehicle_Model_999_Modular_roll_gradient/Inputs/steer_input_selector/Steering Variant Subsystem/sideslip_vs_curvature_1 ==
  Clock : Clock
  Constant : Constant  Value=0
  Constant1 : Constant  Value=steer_input
  Saturation : Saturate  UpperLimit=pi/20
  Switch : Switch  Criteria=u2 > Threshold  Threshold=4  SaturateOnIntegerOverflow=off  InputSameDT=off
  Steer Input : Outport
  wires:
  Switch/1 -> Saturation/1
  Saturation/1 -> Steer Input/1
  Constant1/1 -> Switch/1
  Clock/1 -> Switch/2
  Constant/1 -> Switch/3

== system Vehicle_Model_999_Modular_roll_gradient/Inputs/steer_input_selector/Steering Variant Subsystem/sideslip_vs_curvature_constant_lat_accln ==
  Clock : Clock
  Constant : Constant  Value=0
  Ramp : simulink/Sources/Ramp  slope=pi/100  start=4  InitialOutput=0
  Saturation : Saturate  UpperLimit=pi/20
  Switch : Switch  Criteria=u2 > Threshold  Threshold=4  SaturateOnIntegerOverflow=off  InputSameDT=off
  Steer Input : Outport
  wires:
  Switch/1 -> Saturation/1
  Saturation/1 -> Steer Input/1
  Ramp/1 -> Switch/1
  Clock/1 -> Switch/2
  Constant/1 -> Switch/3

== system Vehicle_Model_999_Modular_roll_gradient/Inputs/steer_input_selector/Steering Variant Subsystem/steerdiff_vs_ay ==
  Clock : Clock
  Constant : Constant  Value=0
  Ramp : simulink/Sources/Ramp  slope=pi/30  start=5  InitialOutput=0
  Saturation : Saturate  UpperLimit=pi/6  LowerLimit=0
  Switch : Switch  Criteria=u2 > Threshold  Threshold=5  SaturateOnIntegerOverflow=off  InputSameDT=off
  Steer Input : Outport
  wires:
  Switch/1 -> Saturation/1
  Ramp/1 -> Switch/1
  Constant/1 -> Switch/3
  Clock/1 -> Switch/2
  Saturation/1 -> Steer Input/1

== system Vehicle_Model_999_Modular_roll_gradient/Vehicle dynamics/Force and Torque Equilibrium/Subsystem/Triggered Subsystem ==
  In1 : Inport
  Trigger : TriggerPort  VariantControl=(inherit)
  Out1 : Outport
  wires:
  In1/1 -> Out1/1

== system Vehicle_Model_999_Modular_roll_gradient/Vehicle dynamics/Fx, Fy calculations/Slip_angle_calculation/Subsystem ==
  toe : Inport
  slip_angles : Inport  Port=2
  Subtract : Sum  Inputs=+-
  slip_ratio : Outport
  wires:
  slip_angles/1 -> Subtract/1
  toe/1 -> Subtract/2
  Subtract/1 -> slip_ratio/1

== system Vehicle_Model_999_Modular_roll_gradient/Vehicle dynamics/Fx, Fy calculations/Slip_angle_calculation/Visualize Slip_angle ==
  slip_angle : Inport
  Demux : Demux
  To Workspace : ToWorkspace  VariableName=slip_angle_fl  SaveFormat=Timeseries  SampleTime=-1
  To Workspace1 : ToWorkspace  VariableName=slip_angle_fr  SaveFormat=Timeseries  SampleTime=-1
  To Workspace2 : ToWorkspace  VariableName=slip_angle_rl  SaveFormat=Timeseries  SampleTime=-1
  To Workspace3 : ToWorkspace  VariableName=slip_angle_rr  SaveFormat=Timeseries  SampleTime=-1
  Visualize_slip_angle : Scope  NumInputPorts=4
      settings: ActiveDisplayYMinimum=-1  ActiveDisplayYMaximum=1  DataLoggingVariableName=ScopeData2
  wires:
  slip_angle/1 -> Demux/1
  Demux/1 -> To Workspace/1, Visualize_slip_angle/1  "slip_angle_fl"
  Demux/2 -> To Workspace1/1, Visualize_slip_angle/2  "slip_angle_fr"
  Demux/3 -> To Workspace2/1, Visualize_slip_angle/3  "slip_angle_rl"
  Demux/4 -> To Workspace3/1, Visualize_slip_angle/4  "slip_angle_rr"

== system Vehicle_Model_999_Modular_roll_gradient/Vehicle dynamics/Fx, Fy calculations/Slip_ratio_calculation/Visualize Slip_ratios ==
  slip_ratio : Inport
  Demux : Demux
  To Workspace : ToWorkspace  VariableName=slip_ratio_fl  SaveFormat=Timeseries  SampleTime=-1
  To Workspace1 : ToWorkspace  VariableName=slip_ratio_fr  SaveFormat=Timeseries  SampleTime=-1
  To Workspace2 : ToWorkspace  VariableName=slip_ratio_rl  SaveFormat=Timeseries  SampleTime=-1
  To Workspace3 : ToWorkspace  VariableName=slip_ratio_rr  SaveFormat=Timeseries  SampleTime=-1
  Visualize_slip_ratio : Scope  NumInputPorts=4
      settings: ActiveDisplayYMinimum=-1  ActiveDisplayYMaximum=1  DataLoggingVariableName=ScopeData2
  wires:
  slip_ratio/1 -> Demux/1
  Demux/1 -> To Workspace/1, Visualize_slip_ratio/1  "slip_ratio_fl"
  Demux/2 -> Visualize_slip_ratio/2, To Workspace1/1  "slip_ratio_fr"
  Demux/3 -> Visualize_slip_ratio/3, To Workspace2/1  "slip_ratio_rl"
  Demux/4 -> Visualize_slip_ratio/4, To Workspace3/1  "slip_ratio_rr"

== system Vehicle_Model_999_Modular_roll_gradient/Vehicle dynamics/Fx, Fy calculations with grip limit/Slip_angle_calculation/Subsystem ==
  toe : Inport
  slip_angles : Inport  Port=2
  Subtract : Sum  Inputs=+-
  slip_ratio : Outport
  wires:
  Subtract/1 -> slip_ratio/1
  toe/1 -> Subtract/2
  slip_angles/1 -> Subtract/1

== system Vehicle_Model_999_Modular_roll_gradient/Vehicle dynamics/Fx, Fy calculations with grip limit/Slip_angle_calculation/Visualize Slip_angle ==
  slip_angle : Inport
  Demux : Demux
  To Workspace : ToWorkspace  VariableName=slip_angle_fl  SaveFormat=Timeseries  SampleTime=-1
  To Workspace1 : ToWorkspace  VariableName=slip_angle_fr  SaveFormat=Timeseries  SampleTime=-1
  To Workspace2 : ToWorkspace  VariableName=slip_angle_rl  SaveFormat=Timeseries  SampleTime=-1
  To Workspace3 : ToWorkspace  VariableName=slip_angle_rr  SaveFormat=Timeseries  SampleTime=-1
  Visualize_slip_angle : Scope  NumInputPorts=4
      settings: ActiveDisplayYMinimum=-1  ActiveDisplayYMaximum=1  DataLoggingVariableName=ScopeData2
  wires:
  Demux/4 -> Visualize_slip_angle/4, To Workspace3/1  "slip_angle_rr"
  Demux/3 -> Visualize_slip_angle/3, To Workspace2/1  "slip_angle_rl"
  Demux/2 -> Visualize_slip_angle/2, To Workspace1/1  "slip_angle_fr"
  Demux/1 -> Visualize_slip_angle/1, To Workspace/1  "slip_angle_fl"
  slip_angle/1 -> Demux/1

== system Vehicle_Model_999_Modular_roll_gradient/Vehicle dynamics/Fx, Fy calculations with grip limit/Slip_ratio_calculation/Visualize Slip_ratios ==
  slip_ratio : Inport
  Demux : Demux
  To Workspace : ToWorkspace  VariableName=slip_ratio_fl  SaveFormat=Timeseries  SampleTime=-1
  To Workspace1 : ToWorkspace  VariableName=slip_ratio_fr  SaveFormat=Timeseries  SampleTime=-1
  To Workspace2 : ToWorkspace  VariableName=slip_ratio_rl  SaveFormat=Timeseries  SampleTime=-1
  To Workspace3 : ToWorkspace  VariableName=slip_ratio_rr  SaveFormat=Timeseries  SampleTime=-1
  Visualize_slip_ratio : Scope  NumInputPorts=4
      settings: ActiveDisplayYMinimum=-1  ActiveDisplayYMaximum=1  DataLoggingVariableName=ScopeData2
  wires:
  Demux/4 -> To Workspace3/1, Visualize_slip_ratio/4  "slip_ratio_rr"
  Demux/3 -> To Workspace2/1, Visualize_slip_ratio/3  "slip_ratio_rl"
  Demux/2 -> To Workspace1/1, Visualize_slip_ratio/2  "slip_ratio_fr"
  Demux/1 -> Visualize_slip_ratio/1, To Workspace/1  "slip_ratio_fl"
  slip_ratio/1 -> Demux/1

== matlab function Vehicle_Model_999_Modular_roll_gradient/Vehicle dynamics/Fx, Fy calculations/Wheel to Vehicle Coordinates ==
  data: Fx_w input; Fx_b output; Fy_w input; Steer_FL input; Steer_FR input; Fy_b output
function [Fx_b, Fy_b] = fcn(Fx_w, Fy_w, Steer_FL, Steer_FR)
%#codegen
% FORCE & MOMENT RESOLVER
    % 1. Construct Steering Vector [FL; FR; RL; RR]
    % Rear steering is assumed to be 0
    Delta = [Steer_FL; Steer_FR; 0; 0];
    
    % 2. Pre-calculate Trig functions (Vectorized)
    c_d = cos(Delta);
    s_d = sin(Delta);
    
    % Longitudinal Body Force:

    Fx_b = Fx_w .* c_d - Fy_w .* s_d;
    
    % Lateral Body Force:
    % Fy_body = Fx_wheel * sin(delta) + Fy_wheel * cos(delta)
    Fy_b = Fx_w .* s_d + Fy_w .* c_d;
    
    % 4. Summation: Total Forces acting on CG
    %B_Fx = sum(Fx_b);
    %B_Fy = sum(Fy_b);
    
end

== matlab function Vehicle_Model_999_Modular_roll_gradient/Vehicle dynamics/Wheel_dynamics/Rolling Resistance ==
  data: Fz input; wFx_rr output; Omega input; slip_angles input; Par parameter
function wFx_rr  = fcn(Fz, Omega,slip_angles, Par)
%#codegen

    % 1. Calculate Total Magnitude
    F_mag = Par.C_rr .* abs(Fz);

    % 2. Determine Direction
    Dir = tanh(10 * Omega);

    
    % X-Component: Resists Spin (Torque generating)
    % wFx = -Magnitude * Direction * cos(Alpha)
    wFx_rr = -F_mag .*Dir.* cos(slip_angles);

end
